simulink model "GPC_DT_ss"  (R2020b)
settings: Solver=VariableStepAuto  StartTime=0.0  StopTime=70  RelTol=1e-3
undefined symbols (not defined in the file): A_ss_DT, D_ss_DT, DT_3, FIR, H_ss_DT, KE_ss_DT, KF_ss_DT, Kr_ss_DT
libraries: cstblocks x1
settings Model: Creator=LACER_GMG  LastModifiedBy=GMG

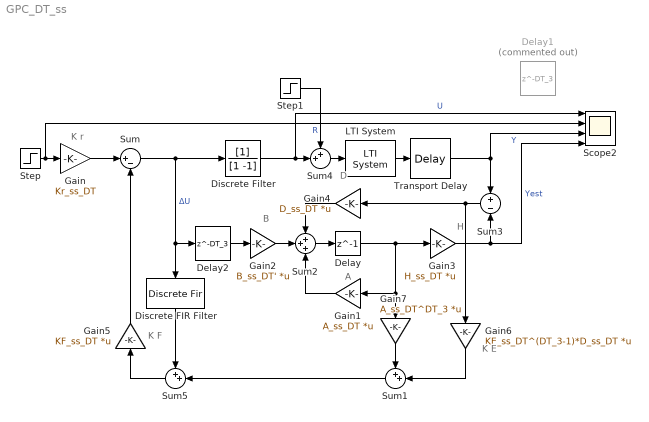
== system GPC_DT_ss ==
  note: D
  note: A
  note: B
  note: K F
  note: K E
  note: H
  note: K r
  Delay : Delay  DelayLength=1  InitialCondition=[0 0]
  Delay1 : Delay  Commented=on  DelayLength=DT_3
  Delay2 : Delay  DelayLength=DT_3
  Discrete FIR Filter : DiscreteFir  Coefficients=FIR
  Discrete Filter : DiscreteFilter  Denominator=[1 -1]  FilterStructure=Direct form I
  Gain : Gain  Gain=Kr_ss_DT
  Gain1 : Gain  Gain=A_ss_DT  Multiplication=Matrix(K*u)
  Gain2 : Gain  Gain=B_ss_DT'  Multiplication=Matrix(K*u)
  Gain3 : Gain  Gain=H_ss_DT  Multiplication=Matrix(K*u)
  Gain4 : Gain  Gain=D_ss_DT  Multiplication=Matrix(K*u)
  Gain5 : Gain  Gain=KF_ss_DT  Multiplication=Matrix(K*u)
  Gain6 : Gain  Gain=KE_ss_DT^(DT_3-1)*D_ss_DT  Multiplication=Matrix(K*u)
  Gain7 : Gain  Gain=A_ss_DT^DT_3  Multiplication=Matrix(K*u)
  LTI System : cstblocks/LTI System  sys=P_ss_DT  IC=[]
  Scope2 : Scope  NumInputPorts=4
  Step : Step  SampleTime=1
  Step1 : Step  Time=25  SampleTime=0
  Sum : Sum  Inputs=|+-
  Sum1 : Sum  Inputs=++|
  Sum2 : Sum  Inputs=+++
  Sum3 : Sum  Inputs=+|-
  Sum4 : Sum  Inputs=++|
  Sum5 : Sum  Inputs=++|
  Transport Delay : TransportDelay  DelayTime=DT_3
  wires:
  Step/1 -> Scope2/2, Gain/1  "R"
  Discrete Filter/1 -> Scope2/1, Sum4/2  "U"
  Gain5/1 -> Sum/2
  Gain2/1 -> Sum2/2
  Sum3/1 -> Gain6/1, Gain4/1
  Gain3/1 -> Scope2/4, Sum3/2  "Yest"
  Delay/1 -> Gain7/1, Gain1/1, Gain3/1
  Gain4/1 -> Sum2/1
  Sum2/1 -> Delay/1
  Gain1/1 -> Sum2/3
  Gain7/1 -> Sum1/1
  Gain6/1 -> Sum1/2
  Gain/1 -> Sum/1
  Sum/1 -> Discrete Filter/1, Delay2/1, Discrete FIR Filter/1  "ΔU"
  Transport Delay/1 -> Scope2/3, Sum3/1  "Y"
  Sum4/1 -> LTI System/1
  Step1/1 -> Sum4/1
  Delay2/1 -> Gain2/1
  Sum1/1 -> Sum5/2
  Discrete FIR Filter/1 -> Sum5/1
  Sum5/1 -> Gain5/1
  LTI System/1 -> Transport Delay/1
